simulink model "DV3A_String1_Diode"  (R2023b)
settings: Solver=VariableStepAuto  StartTime=0.0  StopTime=1  FixedStep=Ts_Power  MinStep=0.0025  RelTol=1e-4
PreLoadFcn:
  | Ts_Power=5e-4;
  | Slope_Vdc=1;
InitFcn:
  | Ts_Power=50e-6;
  | Tc=1e-5;%break algebraic loop time constant
StopFcn:
  | if exist('I','var') && exist('V','var')
  |    figure(1)
  |    clf
  |    n=find(I>=0);
  |    n=n(end);
  |    Vglobal=V(1:n);
  |    Iglobal=I(1:n);
  | 
  | 
  |    Pglobal=Vglobal.*Iglobal;
  |    n=find(Pglobal==max(Pglobal));
  |    Pmax=Pglobal(n);
  |    Vmp=Vglobal(n);
  |    Imp=Iglobal(n);
  | 
  | 
  |    subplot(211)
  |    plot(Vglobal, Iglobal,Vmp,Imp,'or')
  |    ylabel('Current (A)')
  |    title(sprintf('Global I-V & P-V characteristics\n %s' ,ModuleName))
  | 
  | 
  |    subplot(212)
  |    plot(Vglobal, Pglobal,Vmp,Pmax,'or')
  |    ylabel('Power (W)')
  |    xlabel('Voltage (V)')
  | end
model workspace (MAT data in the model file):
  slope_Vdc = 3.0848387096
values from neighbouring files (symbols this model uses):
  Slope_Vdc_string1 = Slope_Vdc_string(1)    [totPower.m]
libraries: spsPVArrayLib x121, spsVariableResistorLib x121, spsDiodeLib x24, spsCurrentMeasurementLib x1, spsVoltageMeasurementLib x1, spsControlledVoltageSourceLib x1, simulink x1, spspowerguiLib x1
(part 1 of 7)
settings Model: Creator=MathWorks  LastModifiedBy=IT
settings SolverCC: AlgebraicLoopSolver=LineSearch
settings DataIOCC: ExternalInput=[]  LimitDataPoints=on  LoadExternalInput=on  SaveFormat=Array  SaveOutput=off  SignalLogging=off  DSMLogging=off  SaveTime=off  ReturnWorkspaceOutputs=off
settings OptimizationCC: ExpressionDepthLimit=2147483647  LifeSpan=inf
settings DebuggingCC: UnderspecifiedInitializationDetection=Classic  MergeDetectMultiDrivingBlocksExec=none  SolverPrmCheckMsg=warning  FcnCallInpInsideContextMsg=warning  UnconnectedInputMsg=warning  UnconnectedOutputMsg=warning  UnconnectedLineMsg=warning  AllowSymbolicDim=off  StateNameClashWarn=warning  SFUnexpectedBacktrackingDiag=warning  SFNoUnconditionalDefaultTransitionDiag=warning  SFExecutionAtInitializationDiag=none  ArithmeticOperatorsInVariantConditions=warning
settings HardwareCC: ProdBitPerPointer=32  ProdBitPerSizeT=32  ProdBitPerPtrDiffT=32  ProdLargestAtomicFloat=None  ProdIntDivRoundTo=Undefined  ProdEndianess=Unspecified  ProdWordSize=32  ProdHWDeviceType=32-bit Generic
settings ModelReferenceCC: EnableRefExpFcnMdlSchedulingChecks=on  PropagateSignalLabelsOutOfModel=off
settings SFSimCC: SimUseLocalCustomCode=off  CustomCodeUndefinedFunction=UseInterfaceOnly
settings RTWCC: RTWUseLocalCustomCode=off  DLArmComputeVersion=19.05
settings CodeAppCC: StateflowObjectComments=on
settings GRTTargetCC: TargetLangStandard=C89/C90 (ANSI)  CombineOutputUpdateFcns=off  GRTInterface=on
settings ConfigComp: CovMetricSettings=dw  CovSaveCumulativeToWorkspaceVar=on  CovSaveSingleToWorkspaceVar=on  CovExternalEMLEnable=off  CovSFcnEnable=off
settings SimscapeCC: SimscapeNormalizeSystem=off

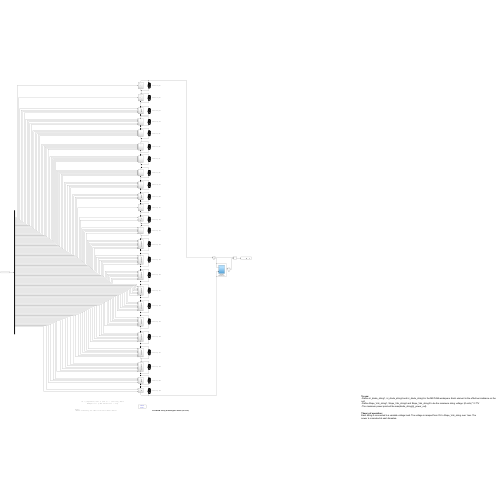
[thumbnail: Simulink's stored preview of the top-level diagram]
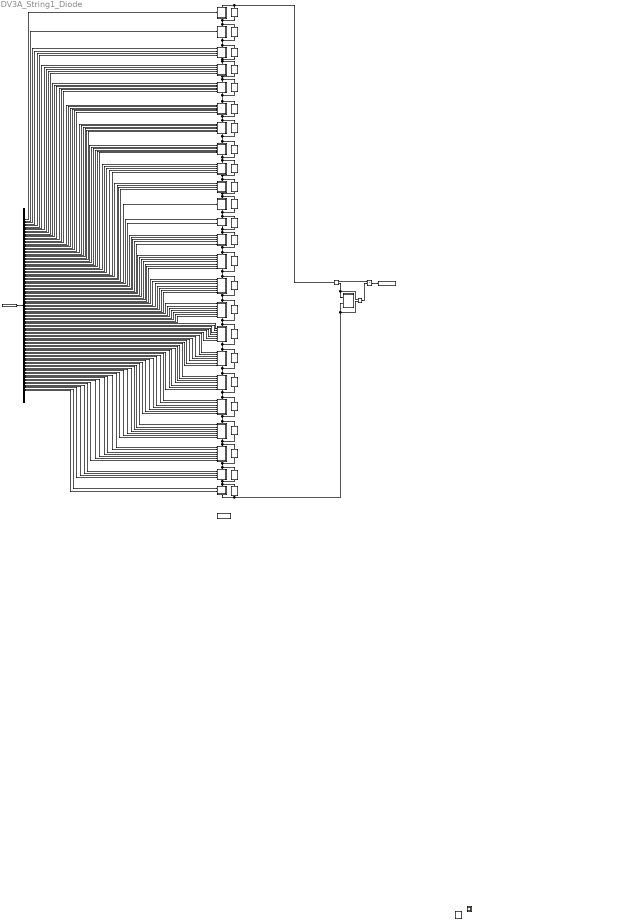
== system DV3A_String1_Diode ==
  note: irr = [(required 0) (cell 1) (cell 2) ... (cell 121)], W/m^2
  note: Notes:
      | -Within a substring, the order of the cells doesn't matter
  note: Final DV3B - String #1 with bypass diodes (121 cells)
  note: Example: irr = [0 800 700 242 573.3 ... 473]
  note: To use:
      | -Define irr_diode_string1, irr_diode_string2 and irr_diode_string3 in the MATLAB workspace. Each element is the effective irradiance on the cell
      | -Define Slope_Vdc_string1, Slope_Vdc_string2 and Slope_Vdc_string3 to be the maximum string voltage: (# cells) * 0.77V
      | -The maximum power point will be max(diode_string[n]_power_out )
  note: Theory of operation:
      | Each string is connected to a variable voltage load. The voltage is ramped from 0V to Slope_Vdc_string over 1sec. The power is computed at each timestep.
  note: Substring #1
  note: Substring #2
  note: Substring #3
  note: Substring #4
  note: Substring #5
  note: Substring #6
  note: Substring #8
  note: Substring #7
  note: Substring #9
  note: Substring #10
  note: Substring #11
  note: Substring #12
  note: Substring #13
  note: Substring #14
  note: Substring #15
  note: Substring #17
  note: Substring #16
  note: Substring #19
  note: Substring #18
  note: Substring #20
  note: Substring #21
  note: Substring #22
  note: Substring #23
  note: Substring #24
  Bypass Diode {1..11,21..33} (24 alike) : spsDiodeLib/Diode  Ron=0.00333333  Lon=0  Vf=0.01993333134  IC=0  UseSnubber=off  Rs=1000000000  Cs=250e-15  Measurements=off
  Demux2 : Demux  Outputs=121
  From Workspace2 : FromWorkspace  VariableName=irr_diode_string_String1
  I1 : spsCurrentMeasurementLib/Current Measurement  PhasorSimulation=off  OutputType=Complex  PSBequivalent=0
  Product2 : Product
  Subsystem1 : Subsystem
      settings: PortSchema="{\"entries\":[{\"content\":{\"sides\":[{\"content\":{\"connectorIds\":[\"In1\",\"In2\",\"In3\",\"In4\",\"In5\",\"In6\",\"In7\"]},\"type\":\"ConnectorPlacement.EquallySpacedRectSide\",\"uuid\":\"ec6071b1-e44d-45a4-9204-34cda7b2c9be\"},{\"content\":{\"connectorIds\":[],\"side\":\"RIGHT\"},\"type\":\"ConnectorPlacement.EquallySpacedRectSide\",\"uuid\":\"8ac2ba72-278d-4942-985d-63a53d830fa7\"},{\"content\":{\"connectorIds\":[\"LConn1\"],\"side\":\"TOP\"},\"type\":\"ConnectorPlacement.EquallySpacedRectSide\",\"uuid\":\"91abef48-6106-4bba-9094-b5b4c6d4927b\"},{\"content\":{\"connectorIds\":[\"RConn1\"],\"side\":\"BOTTOM\"},\"type\":\"ConnectorPlacement.EquallySpacedRectSide\",\"uuid\":\"2339e630-2664-445f-8cd2-24ead5b760e5\"}]},\"type\":\"ConnectorPlacement.EquallySpacedConnector\",\"uuid\":\"6b30c10d-3aac-43c1-96cb-d205f04f2f88\"}],\"packageUris\":[\"http://schema.mathworks.com/mf0/Connector/R2020b\"],\"version\":\"1.0\"}"
  Subsystem10 : Subsystem
      settings: PortSchema="{\"entries\":[{\"content\":{\"sides\":[{\"content\":{\"connectorIds\":[\"In1\",\"In2\",\"In3\",\"In4\"]},\"type\":\"ConnectorPlacement.EquallySpacedRectSide\",\"uuid\":\"ec6071b1-e44d-45a4-9204-34cda7b2c9be\"},{\"content\":{\"connectorIds\":[],\"side\":\"RIGHT\"},\"type\":\"ConnectorPlacement.EquallySpacedRectSide\",\"uuid\":\"8ac2ba72-278d-4942-985d-63a53d830fa7\"},{\"content\":{\"connectorIds\":[\"LConn1\"],\"side\":\"TOP\"},\"type\":\"ConnectorPlacement.EquallySpacedRectSide\",\"uuid\":\"91abef48-6106-4bba-9094-b5b4c6d4927b\"},{\"content\":{\"connectorIds\":[\"RConn1\"],\"side\":\"BOTTOM\"},\"type\":\"ConnectorPlacement.EquallySpacedRectSide\",\"uuid\":\"2339e630-2664-445f-8cd2-24ead5b760e5\"}]},\"type\":\"ConnectorPlacement.EquallySpacedConnector\",\"uuid\":\"6b30c10d-3aac-43c1-96cb-d205f04f2f88\"}],\"packageUris\":[\"http://schema.mathworks.com/mf0/Connector/R2020b\"],\"version\":\"1.0\"}"
  Subsystem11 : Subsystem
      settings: PortSchema="{\"entries\":[{\"content\":{\"sides\":[{\"content\":{\"connectorIds\":[\"In1\",\"In2\"]},\"type\":\"ConnectorPlacement.EquallySpacedRectSide\",\"uuid\":\"ec6071b1-e44d-45a4-9204-34cda7b2c9be\"},{\"content\":{\"connectorIds\":[],\"side\":\"RIGHT\"},\"type\":\"ConnectorPlacement.EquallySpacedRectSide\",\"uuid\":\"8ac2ba72-278d-4942-985d-63a53d830fa7\"},{\"content\":{\"connectorIds\":[\"LConn1\"],\"side\":\"TOP\"},\"type\":\"ConnectorPlacement.EquallySpacedRectSide\",\"uuid\":\"91abef48-6106-4bba-9094-b5b4c6d4927b\"},{\"content\":{\"connectorIds\":[\"RConn1\"],\"side\":\"BOTTOM\"},\"type\":\"ConnectorPlacement.EquallySpacedRectSide\",\"uuid\":\"2339e630-2664-445f-8cd2-24ead5b760e5\"}]},\"type\":\"ConnectorPlacement.EquallySpacedConnector\",\"uuid\":\"6b30c10d-3aac-43c1-96cb-d205f04f2f88\"}],\"packageUris\":[\"http://schema.mathworks.com/mf0/Connector/R2020b\"],\"version\":\"1.0\"}"
  Subsystem2 : Subsystem
      settings: PortSchema="{\"entries\":[{\"content\":{\"sides\":[{\"content\":{\"connectorIds\":[\"In1\",\"In2\",\"In3\",\"In4\",\"In5\",\"In6\",\"In7\"]},\"type\":\"ConnectorPlacement.EquallySpacedRectSide\",\"uuid\":\"ec6071b1-e44d-45a4-9204-34cda7b2c9be\"},{\"content\":{\"connectorIds\":[],\"side\":\"RIGHT\"},\"type\":\"ConnectorPlacement.EquallySpacedRectSide\",\"uuid\":\"8ac2ba72-278d-4942-985d-63a53d830fa7\"},{\"content\":{\"connectorIds\":[\"LConn1\"],\"side\":\"TOP\"},\"type\":\"ConnectorPlacement.EquallySpacedRectSide\",\"uuid\":\"91abef48-6106-4bba-9094-b5b4c6d4927b\"},{\"content\":{\"connectorIds\":[\"RConn1\"],\"side\":\"BOTTOM\"},\"type\":\"ConnectorPlacement.EquallySpacedRectSide\",\"uuid\":\"2339e630-2664-445f-8cd2-24ead5b760e5\"}]},\"type\":\"ConnectorPlacement.EquallySpacedConnector\",\"uuid\":\"6b30c10d-3aac-43c1-96cb-d205f04f2f88\"}],\"packageUris\":[\"http://schema.mathworks.com/mf0/Connector/R2020b\"],\"version\":\"1.0\"}"
  Subsystem21 : Subsystem
      settings: PortSchema="{\"entries\":[{\"content\":{\"sides\":[{\"content\":{\"connectorIds\":[\"In1\"]},\"type\":\"ConnectorPlacement.EquallySpacedRectSide\",\"uuid\":\"ec6071b1-e44d-45a4-9204-34cda7b2c9be\"},{\"content\":{\"side\":\"RIGHT\"},\"type\":\"ConnectorPlacement.EquallySpacedRectSide\",\"uuid\":\"8ac2ba72-278d-4942-985d-63a53d830fa7\"},{\"content\":{\"connectorIds\":[\"LConn1\"],\"side\":\"TOP\"},\"type\":\"ConnectorPlacement.EquallySpacedRectSide\",\"uuid\":\"91abef48-6106-4bba-9094-b5b4c6d4927b\"},{\"content\":{\"connectorIds\":[\"RConn1\"],\"side\":\"BOTTOM\"},\"type\":\"ConnectorPlacement.EquallySpacedRectSide\",\"uuid\":\"2339e630-2664-445f-8cd2-24ead5b760e5\"}]},\"type\":\"ConnectorPlacement.EquallySpacedConnector\",\"uuid\":\"6b30c10d-3aac-43c1-96cb-d205f04f2f88\"}],\"packageUris\":[\"http://schema.mathworks.com/mf0/Connector/R2020b\"],\"version\":\"1.0\"}"
  Subsystem22 : Subsystem
      settings: PortSchema="{\"entries\":[{\"content\":{\"sides\":[{\"content\":{\"connectorIds\":[\"In1\"]},\"type\":\"ConnectorPlacement.EquallySpacedRectSide\",\"uuid\":\"ec6071b1-e44d-45a4-9204-34cda7b2c9be\"},{\"content\":{\"side\":\"RIGHT\"},\"type\":\"ConnectorPlacement.EquallySpacedRectSide\",\"uuid\":\"8ac2ba72-278d-4942-985d-63a53d830fa7\"},{\"content\":{\"connectorIds\":[\"LConn1\"],\"side\":\"TOP\"},\"type\":\"ConnectorPlacement.EquallySpacedRectSide\",\"uuid\":\"91abef48-6106-4bba-9094-b5b4c6d4927b\"},{\"content\":{\"connectorIds\":[\"RConn1\"],\"side\":\"BOTTOM\"},\"type\":\"ConnectorPlacement.EquallySpacedRectSide\",\"uuid\":\"2339e630-2664-445f-8cd2-24ead5b760e5\"}]},\"type\":\"ConnectorPlacement.EquallySpacedConnector\",\"uuid\":\"6b30c10d-3aac-43c1-96cb-d205f04f2f88\"}],\"packageUris\":[\"http://schema.mathworks.com/mf0/Connector/R2020b\"],\"version\":\"1.0\"}"
  Subsystem23 : Subsystem
      settings: PortSchema="{\"entries\":[{\"content\":{\"sides\":[{\"content\":{\"connectorIds\":[\"In1\",\"In2\",\"In3\",\"In4\"]},\"type\":\"ConnectorPlacement.EquallySpacedRectSide\",\"uuid\":\"ec6071b1-e44d-45a4-9204-34cda7b2c9be\"},{\"content\":{\"connectorIds\":[],\"side\":\"RIGHT\"},\"type\":\"ConnectorPlacement.EquallySpacedRectSide\",\"uuid\":\"8ac2ba72-278d-4942-985d-63a53d830fa7\"},{\"content\":{\"connectorIds\":[\"LConn1\"],\"side\":\"TOP\"},\"type\":\"ConnectorPlacement.EquallySpacedRectSide\",\"uuid\":\"91abef48-6106-4bba-9094-b5b4c6d4927b\"},{\"content\":{\"connectorIds\":[\"RConn1\"],\"side\":\"BOTTOM\"},\"type\":\"ConnectorPlacement.EquallySpacedRectSide\",\"uuid\":\"2339e630-2664-445f-8cd2-24ead5b760e5\"}]},\"type\":\"ConnectorPlacement.EquallySpacedConnector\",\"uuid\":\"6b30c10d-3aac-43c1-96cb-d205f04f2f88\"}],\"packageUris\":[\"http://schema.mathworks.com/mf0/Connector/R2020b\"],\"version\":\"1.0\"}"
  Subsystem24 : Subsystem
      settings: PortSchema="{\"entries\":[{\"content\":{\"sides\":[{\"content\":{\"connectorIds\":[\"In1\",\"In2\",\"In3\",\"In4\",\"In5\"]},\"type\":\"ConnectorPlacement.EquallySpacedRectSide\",\"uuid\":\"ec6071b1-e44d-45a4-9204-34cda7b2c9be\"},{\"content\":{\"side\":\"RIGHT\"},\"type\":\"ConnectorPlacement.EquallySpacedRectSide\",\"uuid\":\"8ac2ba72-278d-4942-985d-63a53d830fa7\"},{\"content\":{\"connectorIds\":[\"LConn1\"],\"side\":\"TOP\"},\"type\":\"ConnectorPlacement.EquallySpacedRectSide\",\"uuid\":\"91abef48-6106-4bba-9094-b5b4c6d4927b\"},{\"content\":{\"connectorIds\":[\"RConn1\"],\"side\":\"BOTTOM\"},\"type\":\"ConnectorPlacement.EquallySpacedRectSide\",\"uuid\":\"2339e630-2664-445f-8cd2-24ead5b760e5\"}]},\"type\":\"ConnectorPlacement.EquallySpacedConnector\",\"uuid\":\"6b30c10d-3aac-43c1-96cb-d205f04f2f88\"}],\"packageUris\":[\"http://schema.mathworks.com/mf0/Connector/R2020b\"],\"version\":\"1.0\"}"
  Subsystem25 : Subsystem
      settings: PortSchema="{\"entries\":[{\"content\":{\"sides\":[{\"content\":{\"connectorIds\":[\"In1\",\"In2\",\"In3\",\"In4\",\"In5\",\"In6\"]},\"type\":\"ConnectorPlacement.EquallySpacedRectSide\",\"uuid\":\"ec6071b1-e44d-45a4-9204-34cda7b2c9be\"},{\"content\":{\"side\":\"RIGHT\"},\"type\":\"ConnectorPlacement.EquallySpacedRectSide\",\"uuid\":\"8ac2ba72-278d-4942-985d-63a53d830fa7\"},{\"content\":{\"connectorIds\":[\"LConn1\"],\"side\":\"TOP\"},\"type\":\"ConnectorPlacement.EquallySpacedRectSide\",\"uuid\":\"91abef48-6106-4bba-9094-b5b4c6d4927b\"},{\"content\":{\"connectorIds\":[\"RConn1\"],\"side\":\"BOTTOM\"},\"type\":\"ConnectorPlacement.EquallySpacedRectSide\",\"uuid\":\"2339e630-2664-445f-8cd2-24ead5b760e5\"}]},\"type\":\"ConnectorPlacement.EquallySpacedConnector\",\"uuid\":\"6b30c10d-3aac-43c1-96cb-d205f04f2f88\"}],\"packageUris\":[\"http://schema.mathworks.com/mf0/Connector/R2020b\"],\"version\":\"1.0\"}"
  Subsystem26 : Subsystem
      settings: PortSchema="{\"entries\":[{\"content\":{\"sides\":[{\"content\":{\"connectorIds\":[\"In1\",\"In2\",\"In3\",\"In4\",\"In5\",\"In6\"]},\"type\":\"ConnectorPlacement.EquallySpacedRectSide\",\"uuid\":\"ec6071b1-e44d-45a4-9204-34cda7b2c9be\"},{\"content\":{\"side\":\"RIGHT\"},\"type\":\"ConnectorPlacement.EquallySpacedRectSide\",\"uuid\":\"8ac2ba72-278d-4942-985d-63a53d830fa7\"},{\"content\":{\"connectorIds\":[\"LConn1\"],\"side\":\"TOP\"},\"type\":\"ConnectorPlacement.EquallySpacedRectSide\",\"uuid\":\"91abef48-6106-4bba-9094-b5b4c6d4927b\"},{\"content\":{\"connectorIds\":[\"RConn1\"],\"side\":\"BOTTOM\"},\"type\":\"ConnectorPlacement.EquallySpacedRectSide\",\"uuid\":\"2339e630-2664-445f-8cd2-24ead5b760e5\"}]},\"type\":\"ConnectorPlacement.EquallySpacedConnector\",\"uuid\":\"6b30c10d-3aac-43c1-96cb-d205f04f2f88\"}],\"packageUris\":[\"http://schema.mathworks.com/mf0/Connector/R2020b\"],\"version\":\"1.0\"}"
  Subsystem27 : Subsystem
      settings: PortSchema="{\"entries\":[{\"content\":{\"sides\":[{\"content\":{\"connectorIds\":[\"In1\",\"In2\",\"In3\",\"In4\",\"In5\",\"In6\"]},\"type\":\"ConnectorPlacement.EquallySpacedRectSide\",\"uuid\":\"ec6071b1-e44d-45a4-9204-34cda7b2c9be\"},{\"content\":{\"side\":\"RIGHT\"},\"type\":\"ConnectorPlacement.EquallySpacedRectSide\",\"uuid\":\"8ac2ba72-278d-4942-985d-63a53d830fa7\"},{\"content\":{\"connectorIds\":[\"LConn1\"],\"side\":\"TOP\"},\"type\":\"ConnectorPlacement.EquallySpacedRectSide\",\"uuid\":\"91abef48-6106-4bba-9094-b5b4c6d4927b\"},{\"content\":{\"connectorIds\":[\"RConn1\"],\"side\":\"BOTTOM\"},\"type\":\"ConnectorPlacement.EquallySpacedRectSide\",\"uuid\":\"2339e630-2664-445f-8cd2-24ead5b760e5\"}]},\"type\":\"ConnectorPlacement.EquallySpacedConnector\",\"uuid\":\"6b30c10d-3aac-43c1-96cb-d205f04f2f88\"}],\"packageUris\":[\"http://schema.mathworks.com/mf0/Connector/R2020b\"],\"version\":\"1.0\"}"
  Subsystem28 : Subsystem
      settings: PortSchema="{\"entries\":[{\"content\":{\"sides\":[{\"content\":{\"connectorIds\":[\"In1\",\"In2\",\"In3\",\"In4\",\"In5\"]},\"type\":\"ConnectorPlacement.EquallySpacedRectSide\",\"uuid\":\"ec6071b1-e44d-45a4-9204-34cda7b2c9be\"},{\"content\":{\"side\":\"RIGHT\"},\"type\":\"ConnectorPlacement.EquallySpacedRectSide\",\"uuid\":\"8ac2ba72-278d-4942-985d-63a53d830fa7\"},{\"content\":{\"connectorIds\":[\"LConn1\"],\"side\":\"TOP\"},\"type\":\"ConnectorPlacement.EquallySpacedRectSide\",\"uuid\":\"91abef48-6106-4bba-9094-b5b4c6d4927b\"},{\"content\":{\"connectorIds\":[\"RConn1\"],\"side\":\"BOTTOM\"},\"type\":\"ConnectorPlacement.EquallySpacedRectSide\",\"uuid\":\"2339e630-2664-445f-8cd2-24ead5b760e5\"}]},\"type\":\"ConnectorPlacement.EquallySpacedConnector\",\"uuid\":\"6b30c10d-3aac-43c1-96cb-d205f04f2f88\"}],\"packageUris\":[\"http://schema.mathworks.com/mf0/Connector/R2020b\"],\"version\":\"1.0\"}"
  Subsystem29 : Subsystem
      settings: PortSchema="{\"entries\":[{\"content\":{\"sides\":[{\"content\":{\"connectorIds\":[\"In1\",\"In2\",\"In3\",\"In4\",\"In5\",\"In6\"]},\"type\":\"ConnectorPlacement.EquallySpacedRectSide\",\"uuid\":\"ec6071b1-e44d-45a4-9204-34cda7b2c9be\"},{\"content\":{\"side\":\"RIGHT\"},\"type\":\"ConnectorPlacement.EquallySpacedRectSide\",\"uuid\":\"8ac2ba72-278d-4942-985d-63a53d830fa7\"},{\"content\":{\"connectorIds\":[\"LConn1\"],\"side\":\"TOP\"},\"type\":\"ConnectorPlacement.EquallySpacedRectSide\",\"uuid\":\"91abef48-6106-4bba-9094-b5b4c6d4927b\"},{\"content\":{\"connectorIds\":[\"RConn1\"],\"side\":\"BOTTOM\"},\"type\":\"ConnectorPlacement.EquallySpacedRectSide\",\"uuid\":\"2339e630-2664-445f-8cd2-24ead5b760e5\"}]},\"type\":\"ConnectorPlacement.EquallySpacedConnector\",\"uuid\":\"6b30c10d-3aac-43c1-96cb-d205f04f2f88\"}],\"packageUris\":[\"http://schema.mathworks.com/mf0/Connector/R2020b\"],\"version\":\"1.0\"}"
  Subsystem3 : Subsystem
      settings: PortSchema="{\"entries\":[{\"content\":{\"sides\":[{\"content\":{\"connectorIds\":[\"In1\",\"In2\",\"In3\",\"In4\",\"In5\",\"In6\",\"In7\"]},\"type\":\"ConnectorPlacement.EquallySpacedRectSide\",\"uuid\":\"ec6071b1-e44d-45a4-9204-34cda7b2c9be\"},{\"content\":{\"connectorIds\":[],\"side\":\"RIGHT\"},\"type\":\"ConnectorPlacement.EquallySpacedRectSide\",\"uuid\":\"8ac2ba72-278d-4942-985d-63a53d830fa7\"},{\"content\":{\"connectorIds\":[\"LConn1\"],\"side\":\"TOP\"},\"type\":\"ConnectorPlacement.EquallySpacedRectSide\",\"uuid\":\"91abef48-6106-4bba-9094-b5b4c6d4927b\"},{\"content\":{\"connectorIds\":[\"RConn1\"],\"side\":\"BOTTOM\"},\"type\":\"ConnectorPlacement.EquallySpacedRectSide\",\"uuid\":\"2339e630-2664-445f-8cd2-24ead5b760e5\"}]},\"type\":\"ConnectorPlacement.EquallySpacedConnector\",\"uuid\":\"6b30c10d-3aac-43c1-96cb-d205f04f2f88\"}],\"packageUris\":[\"http://schema.mathworks.com/mf0/Connector/R2020b\"],\"version\":\"1.0\"}"
  Subsystem30 : Subsystem
      settings: PortSchema="{\"entries\":[{\"content\":{\"sides\":[{\"content\":{\"connectorIds\":[\"In1\",\"In2\",\"In3\",\"In4\"]},\"type\":\"ConnectorPlacement.EquallySpacedRectSide\",\"uuid\":\"ec6071b1-e44d-45a4-9204-34cda7b2c9be\"},{\"content\":{\"connectorIds\":[],\"side\":\"RIGHT\"},\"type\":\"ConnectorPlacement.EquallySpacedRectSide\",\"uuid\":\"8ac2ba72-278d-4942-985d-63a53d830fa7\"},{\"content\":{\"connectorIds\":[\"LConn1\"],\"side\":\"TOP\"},\"type\":\"ConnectorPlacement.EquallySpacedRectSide\",\"uuid\":\"91abef48-6106-4bba-9094-b5b4c6d4927b\"},{\"content\":{\"connectorIds\":[\"RConn1\"],\"side\":\"BOTTOM\"},\"type\":\"ConnectorPlacement.EquallySpacedRectSide\",\"uuid\":\"2339e630-2664-445f-8cd2-24ead5b760e5\"}]},\"type\":\"ConnectorPlacement.EquallySpacedConnector\",\"uuid\":\"6b30c10d-3aac-43c1-96cb-d205f04f2f88\"}],\"packageUris\":[\"http://schema.mathworks.com/mf0/Connector/R2020b\"],\"version\":\"1.0\"}"
  Subsystem31 : Subsystem
      settings: PortSchema="{\"entries\":[{\"content\":{\"sides\":[{\"content\":{\"connectorIds\":[\"In1\"]},\"type\":\"ConnectorPlacement.EquallySpacedRectSide\",\"uuid\":\"ec6071b1-e44d-45a4-9204-34cda7b2c9be\"},{\"content\":{\"side\":\"RIGHT\"},\"type\":\"ConnectorPlacement.EquallySpacedRectSide\",\"uuid\":\"8ac2ba72-278d-4942-985d-63a53d830fa7\"},{\"content\":{\"connectorIds\":[\"LConn1\"],\"side\":\"TOP\"},\"type\":\"ConnectorPlacement.EquallySpacedRectSide\",\"uuid\":\"91abef48-6106-4bba-9094-b5b4c6d4927b\"},{\"content\":{\"connectorIds\":[\"RConn1\"],\"side\":\"BOTTOM\"},\"type\":\"ConnectorPlacement.EquallySpacedRectSide\",\"uuid\":\"2339e630-2664-445f-8cd2-24ead5b760e5\"}]},\"type\":\"ConnectorPlacement.EquallySpacedConnector\",\"uuid\":\"6b30c10d-3aac-43c1-96cb-d205f04f2f88\"}],\"packageUris\":[\"http://schema.mathworks.com/mf0/Connector/R2020b\"],\"version\":\"1.0\"}"
  Subsystem32 : Subsystem
      settings: PortSchema="{\"entries\":[{\"content\":{\"sides\":[{\"content\":{\"connectorIds\":[\"In1\",\"In2\"]},\"type\":\"ConnectorPlacement.EquallySpacedRectSide\",\"uuid\":\"ec6071b1-e44d-45a4-9204-34cda7b2c9be\"},{\"content\":{\"connectorIds\":[],\"side\":\"RIGHT\"},\"type\":\"ConnectorPlacement.EquallySpacedRectSide\",\"uuid\":\"8ac2ba72-278d-4942-985d-63a53d830fa7\"},{\"content\":{\"connectorIds\":[\"LConn1\"],\"side\":\"TOP\"},\"type\":\"ConnectorPlacement.EquallySpacedRectSide\",\"uuid\":\"91abef48-6106-4bba-9094-b5b4c6d4927b\"},{\"content\":{\"connectorIds\":[\"RConn1\"],\"side\":\"BOTTOM\"},\"type\":\"ConnectorPlacement.EquallySpacedRectSide\",\"uuid\":\"2339e630-2664-445f-8cd2-24ead5b760e5\"}]},\"type\":\"ConnectorPlacement.EquallySpacedConnector\",\"uuid\":\"6b30c10d-3aac-43c1-96cb-d205f04f2f88\"}],\"packageUris\":[\"http://schema.mathworks.com/mf0/Connector/R2020b\"],\"version\":\"1.0\"}"
  Subsystem33 : Subsystem
      settings: PortSchema="{\"entries\":[{\"content\":{\"sides\":[{\"content\":{\"connectorIds\":[\"In1\",\"In2\",\"In3\",\"In4\",\"In5\"]},\"type\":\"ConnectorPlacement.EquallySpacedRectSide\",\"uuid\":\"ec6071b1-e44d-45a4-9204-34cda7b2c9be\"},{\"content\":{\"side\":\"RIGHT\"},\"type\":\"ConnectorPlacement.EquallySpacedRectSide\",\"uuid\":\"8ac2ba72-278d-4942-985d-63a53d830fa7\"},{\"content\":{\"connectorIds\":[\"LConn1\"],\"side\":\"TOP\"},\"type\":\"ConnectorPlacement.EquallySpacedRectSide\",\"uuid\":\"91abef48-6106-4bba-9094-b5b4c6d4927b\"},{\"content\":{\"connectorIds\":[\"RConn1\"],\"side\":\"BOTTOM\"},\"type\":\"ConnectorPlacement.EquallySpacedRectSide\",\"uuid\":\"2339e630-2664-445f-8cd2-24ead5b760e5\"}]},\"type\":\"ConnectorPlacement.EquallySpacedConnector\",\"uuid\":\"6b30c10d-3aac-43c1-96cb-d205f04f2f88\"}],\"packageUris\":[\"http://schema.mathworks.com/mf0/Connector/R2020b\"],\"version\":\"1.0\"}"
  Subsystem4 : Subsystem
      settings: PortSchema="{\"entries\":[{\"content\":{\"sides\":[{\"content\":{\"connectorIds\":[\"In1\",\"In2\",\"In3\",\"In4\",\"In5\",\"In6\",\"In7\"]},\"type\":\"ConnectorPlacement.EquallySpacedRectSide\",\"uuid\":\"ec6071b1-e44d-45a4-9204-34cda7b2c9be\"},{\"content\":{\"connectorIds\":[],\"side\":\"RIGHT\"},\"type\":\"ConnectorPlacement.EquallySpacedRectSide\",\"uuid\":\"8ac2ba72-278d-4942-985d-63a53d830fa7\"},{\"content\":{\"connectorIds\":[\"LConn1\"],\"side\":\"TOP\"},\"type\":\"ConnectorPlacement.EquallySpacedRectSide\",\"uuid\":\"91abef48-6106-4bba-9094-b5b4c6d4927b\"},{\"content\":{\"connectorIds\":[\"RConn1\"],\"side\":\"BOTTOM\"},\"type\":\"ConnectorPlacement.EquallySpacedRectSide\",\"uuid\":\"2339e630-2664-445f-8cd2-24ead5b760e5\"}]},\"type\":\"ConnectorPlacement.EquallySpacedConnector\",\"uuid\":\"6b30c10d-3aac-43c1-96cb-d205f04f2f88\"}],\"packageUris\":[\"http://schema.mathworks.com/mf0/Connector/R2020b\"],\"version\":\"1.0\"}"
  Subsystem5 : Subsystem
      settings: PortSchema="{\"entries\":[{\"content\":{\"sides\":[{\"content\":{\"connectorIds\":[\"In1\",\"In2\",\"In3\",\"In4\",\"In5\",\"In6\",\"In7\"]},\"type\":\"ConnectorPlacement.EquallySpacedRectSide\",\"uuid\":\"ec6071b1-e44d-45a4-9204-34cda7b2c9be\"},{\"content\":{\"connectorIds\":[],\"side\":\"RIGHT\"},\"type\":\"ConnectorPlacement.EquallySpacedRectSide\",\"uuid\":\"8ac2ba72-278d-4942-985d-63a53d830fa7\"},{\"content\":{\"connectorIds\":[\"LConn1\"],\"side\":\"TOP\"},\"type\":\"ConnectorPlacement.EquallySpacedRectSide\",\"uuid\":\"91abef48-6106-4bba-9094-b5b4c6d4927b\"},{\"content\":{\"connectorIds\":[\"RConn1\"],\"side\":\"BOTTOM\"},\"type\":\"ConnectorPlacement.EquallySpacedRectSide\",\"uuid\":\"2339e630-2664-445f-8cd2-24ead5b760e5\"}]},\"type\":\"ConnectorPlacement.EquallySpacedConnector\",\"uuid\":\"6b30c10d-3aac-43c1-96cb-d205f04f2f88\"}],\"packageUris\":[\"http://schema.mathworks.com/mf0/Connector/R2020b\"],\"version\":\"1.0\"}"
  Subsystem6 : Subsystem
      settings: PortSchema="{\"entries\":[{\"content\":{\"sides\":[{\"content\":{\"connectorIds\":[\"In1\",\"In2\",\"In3\",\"In4\",\"In5\",\"In6\",\"In7\"]},\"type\":\"ConnectorPlacement.EquallySpacedRectSide\",\"uuid\":\"ec6071b1-e44d-45a4-9204-34cda7b2c9be\"},{\"content\":{\"connectorIds\":[],\"side\":\"RIGHT\"},\"type\":\"ConnectorPlacement.EquallySpacedRectSide\",\"uuid\":\"8ac2ba72-278d-4942-985d-63a53d830fa7\"},{\"content\":{\"connectorIds\":[\"LConn1\"],\"side\":\"TOP\"},\"type\":\"ConnectorPlacement.EquallySpacedRectSide\",\"uuid\":\"91abef48-6106-4bba-9094-b5b4c6d4927b\"},{\"content\":{\"connectorIds\":[\"RConn1\"],\"side\":\"BOTTOM\"},\"type\":\"ConnectorPlacement.EquallySpacedRectSide\",\"uuid\":\"2339e630-2664-445f-8cd2-24ead5b760e5\"}]},\"type\":\"ConnectorPlacement.EquallySpacedConnector\",\"uuid\":\"6b30c10d-3aac-43c1-96cb-d205f04f2f88\"}],\"packageUris\":[\"http://schema.mathworks.com/mf0/Connector/R2020b\"],\"version\":\"1.0\"}"
  Subsystem7 : Subsystem
      settings: PortSchema="{\"entries\":[{\"content\":{\"sides\":[{\"content\":{\"connectorIds\":[\"In1\",\"In2\",\"In3\",\"In4\",\"In5\",\"In6\",\"In7\"]},\"type\":\"ConnectorPlacement.EquallySpacedRectSide\",\"uuid\":\"ec6071b1-e44d-45a4-9204-34cda7b2c9be\"},{\"content\":{\"connectorIds\":[],\"side\":\"RIGHT\"},\"type\":\"ConnectorPlacement.EquallySpacedRectSide\",\"uuid\":\"8ac2ba72-278d-4942-985d-63a53d830fa7\"},{\"content\":{\"connectorIds\":[\"LConn1\"],\"side\":\"TOP\"},\"type\":\"ConnectorPlacement.EquallySpacedRectSide\",\"uuid\":\"91abef48-6106-4bba-9094-b5b4c6d4927b\"},{\"content\":{\"connectorIds\":[\"RConn1\"],\"side\":\"BOTTOM\"},\"type\":\"ConnectorPlacement.EquallySpacedRectSide\",\"uuid\":\"2339e630-2664-445f-8cd2-24ead5b760e5\"}]},\"type\":\"ConnectorPlacement.EquallySpacedConnector\",\"uuid\":\"6b30c10d-3aac-43c1-96cb-d205f04f2f88\"}],\"packageUris\":[\"http://schema.mathworks.com/mf0/Connector/R2020b\"],\"version\":\"1.0\"}"
  Subsystem8 : Subsystem
      settings: PortSchema="{\"entries\":[{\"content\":{\"sides\":[{\"content\":{\"connectorIds\":[\"In1\",\"In2\",\"In3\",\"In4\",\"In5\",\"In6\",\"In7\"]},\"type\":\"ConnectorPlacement.EquallySpacedRectSide\",\"uuid\":\"ec6071b1-e44d-45a4-9204-34cda7b2c9be\"},{\"content\":{\"connectorIds\":[],\"side\":\"RIGHT\"},\"type\":\"ConnectorPlacement.EquallySpacedRectSide\",\"uuid\":\"8ac2ba72-278d-4942-985d-63a53d830fa7\"},{\"content\":{\"connectorIds\":[\"LConn1\"],\"side\":\"TOP\"},\"type\":\"ConnectorPlacement.EquallySpacedRectSide\",\"uuid\":\"91abef48-6106-4bba-9094-b5b4c6d4927b\"},{\"content\":{\"connectorIds\":[\"RConn1\"],\"side\":\"BOTTOM\"},\"type\":\"ConnectorPlacement.EquallySpacedRectSide\",\"uuid\":\"2339e630-2664-445f-8cd2-24ead5b760e5\"}]},\"type\":\"ConnectorPlacement.EquallySpacedConnector\",\"uuid\":\"6b30c10d-3aac-43c1-96cb-d205f04f2f88\"}],\"packageUris\":[\"http://schema.mathworks.com/mf0/Connector/R2020b\"],\"version\":\"1.0\"}"
  Subsystem9 : Subsystem
      settings: PortSchema="{\"entries\":[{\"content\":{\"sides\":[{\"content\":{\"connectorIds\":[\"In1\",\"In2\",\"In3\",\"In4\",\"In5\",\"In6\",\"In7\"]},\"type\":\"ConnectorPlacement.EquallySpacedRectSide\",\"uuid\":\"ec6071b1-e44d-45a4-9204-34cda7b2c9be\"},{\"content\":{\"connectorIds\":[],\"side\":\"RIGHT\"},\"type\":\"ConnectorPlacement.EquallySpacedRectSide\",\"uuid\":\"8ac2ba72-278d-4942-985d-63a53d830fa7\"},{\"content\":{\"connectorIds\":[\"LConn1\"],\"side\":\"TOP\"},\"type\":\"ConnectorPlacement.EquallySpacedRectSide\",\"uuid\":\"91abef48-6106-4bba-9094-b5b4c6d4927b\"},{\"content\":{\"connectorIds\":[\"RConn1\"],\"side\":\"BOTTOM\"},\"type\":\"ConnectorPlacement.EquallySpacedRectSide\",\"uuid\":\"2339e630-2664-445f-8cd2-24ead5b760e5\"}]},\"type\":\"ConnectorPlacement.EquallySpacedConnector\",\"uuid\":\"6b30c10d-3aac-43c1-96cb-d205f04f2f88\"}],\"packageUris\":[\"http://schema.mathworks.com/mf0/Connector/R2020b\"],\"version\":\"1.0\"}"
  To Workspace2 : ToWorkspace  VariableName=diode_string1_power_out  SampleTime=-1
      settings: Save2DSignal=2-D array (concatenate along first dimension)
  V1 : spsVoltageMeasurementLib/Voltage Measurement  PhasorSimulation=off  OutputType=Complex  PSBequivalent=0
  Variable DC Source1 : Subsystem
  powergui2 : spspowerguiLib/powergui  Priority=1  SimulationMode=Discrete  SampleTime=2.5e-3  frequency=60  Iterations=500  frequencyindice=0  Pbase=100e6  ErrMax=1e-4  UnitsV=kV  UnitsW=MW  buscounter=0  FunctionMessages=off  echomessages=off  EnableUseOfTLC=off  CurrentSourceSwitches=on  DisableSnubberDevices=on  DisableRonSwitches=off  DisableVfSwitches=off  DisplayEquations=off  AutomaticDiscreteSolvers=off  SolverType=Tustin/Backward Euler (TBE)  Interpol=off  ExternalGateDelay=off  methode=off  Ts=0  x0status=blocks  SPID=off  SwTol=0  HookPort=off  NonlinearTolerance=1e-4  nMaxIteration=1000  ContinueOnMaxIteration=off  RestoreLinks=warning  ResistiveCurrentMeasurement=off  Frange=[0:2:500]  Ylog=off  Xlog=on  ShowGrid=off  save=off  variable=ZData  structure=0  ZoomFFT=on  StartTime=0.0  cycles=1  DisplayStyle=1  fundamental=60  FreqAxis=off  MaxFrequency=1000  frequencyindicesteady=1  RmsSteady=1  display=off
  Array Plot : ArrayPlot  IOType=viewer  WindowPosition=[117.000000,351.000000,800.000000,450.000000,]  ScopeFrameLocation=window  AxesScaling=Manual  YLimits=[-1,1]
  Scope{,1..3} (4 alike) : Scope
  wires:
  V1/1 -> Product2/2
  Product2/1 -> To Workspace2/1
  I1/1 -> Product2/1
  From Workspace2/1 -> Demux2/1
  Demux2/1 -> Subsystem21/1(Irr)
  Demux2/2 -> Subsystem22/1(Irr)
  Demux2/3 -> Subsystem23/1(Irr)
  Demux2/4 -> Subsystem23/2(Irr1)
  Demux2/5 -> Subsystem23/3(Irr2)
  Demux2/6 -> Subsystem23/4(Irr3)
  Demux2/7 -> Subsystem24/1(Irr)
  Demux2/8 -> Subsystem24/2(Irr1)
  Demux2/9 -> Subsystem24/3(Irr2)
  Demux2/10 -> Subsystem24/4(Irr3)
  Demux2/11 -> Subsystem24/5(Irr4)
  Demux2/12 -> Subsystem29/1(Irr)
  Demux2/13 -> Subsystem29/2(Irr1)
  Demux2/14 -> Subsystem29/3(Irr3)
  Demux2/15 -> Subsystem29/4(Irr4)
  Demux2/16 -> Subsystem29/5(Irr2)
  Demux2/17 -> Subsystem29/6(Irr5)
  Demux2/18 -> Subsystem25/1(Irr)
  Demux2/19 -> Subsystem25/2(Irr1)
  Demux2/20 -> Subsystem25/3(Irr3)
  Demux2/21 -> Subsystem25/4(Irr4)
  Demux2/22 -> Subsystem25/5(Irr2)
  Demux2/23 -> Subsystem25/6(Irr5)
  Demux2/24 -> Subsystem27/1(Irr)
  Demux2/25 -> Subsystem27/2(Irr1)
  Demux2/26 -> Subsystem27/3(Irr3)
  Demux2/28 -> Subsystem27/5(Irr2)
  Demux2/27 -> Subsystem27/4(Irr4)
  Demux2/29 -> Subsystem27/6(Irr5)
  Demux2/30 -> Subsystem26/1(Irr)
  Demux2/31 -> Subsystem26/2(Irr1)
  Demux2/32 -> Subsystem26/3(Irr3)
  Demux2/33 -> Subsystem26/4(Irr4)
  Demux2/34 -> Subsystem26/5(Irr2)
  Demux2/35 -> Subsystem26/6(Irr5)
  Demux2/36 -> Subsystem28/1(Irr)
  Demux2/37 -> Subsystem28/2(Irr1)
  Demux2/38 -> Subsystem28/3(Irr2)
  Demux2/39 -> Subsystem28/4(Irr3)
  Demux2/40 -> Subsystem28/5(Irr4)
  Demux2/41 -> Subsystem30/1(Irr)
  Demux2/42 -> Subsystem30/2(Irr1)
  Demux2/43 -> Subsystem30/3(Irr2)
  Demux2/44 -> Subsystem30/4(Irr3)
  Demux2/45 -> Subsystem31/1(Irr)
  Demux2/46 -> Subsystem32/1(Irr)
  Demux2/47 -> Subsystem32/2(Irr1)
  Demux2/48 -> Subsystem33/1(Irr)
  Demux2/49 -> Subsystem33/2(Irr1)
  Demux2/50 -> Subsystem33/3(Irr2)
  Demux2/51 -> Subsystem33/4(Irr3)
  Demux2/52 -> Subsystem33/5(Irr4)
  Demux2/53 -> Subsystem1/1(Irr)
  Demux2/54 -> Subsystem1/2(Irr1)
  Demux2/55 -> Subsystem1/3(Irr2)
  Demux2/56 -> Subsystem1/4(Irr3)
  Demux2/57 -> Subsystem1/5(Irr4)
  Demux2/58 -> Subsystem1/6(Irr5)
  Demux2/59 -> Subsystem1/7(Irr6)
  Demux2/60 -> Subsystem2/1(Irr)
  Demux2/61 -> Subsystem2/2(Irr1)
  Demux2/62 -> Subsystem2/3(Irr2)
  Demux2/63 -> Subsystem2/4(Irr3)
  Demux2/64 -> Subsystem2/5(Irr4)
  Demux2/65 -> Subsystem2/6(Irr5)
  Demux2/66 -> Subsystem2/7(Irr6)
  Demux2/67 -> Subsystem3/1(Irr)
  Demux2/68 -> Subsystem3/2(Irr1)
  Demux2/69 -> Subsystem3/3(Irr2)
  Demux2/70 -> Subsystem3/4(Irr3)
  Demux2/71 -> Subsystem3/5(Irr4)
  Demux2/72 -> Subsystem3/6(Irr5)
  Demux2/73 -> Subsystem3/7(Irr6)
  Demux2/74 -> Subsystem4/1(Irr)
  Demux2/75 -> Subsystem4/2(Irr1)
  Demux2/76 -> Subsystem4/3(Irr2)
  Demux2/77 -> Subsystem4/4(Irr3)
  Demux2/78 -> Subsystem4/5(Irr4)
  Demux2/79 -> Subsystem4/6(Irr5)
  Demux2/80 -> Subsystem4/7(Irr6)
  Demux2/81 -> Subsystem5/1(Irr)
  Demux2/82 -> Subsystem5/2(Irr1)
  Demux2/83 -> Subsystem5/3(Irr2)
  Demux2/84 -> Subsystem5/4(Irr3)
  Demux2/85 -> Subsystem5/5(Irr4)
  Demux2/86 -> Subsystem5/6(Irr5)
  Demux2/87 -> Subsystem5/7(Irr6)
  Demux2/88 -> Subsystem6/1(Irr)
  Demux2/89 -> Subsystem6/2(Irr1)
  Demux2/90 -> Subsystem6/3(Irr2)
  Demux2/91 -> Subsystem6/4(Irr3)
  Demux2/92 -> Subsystem6/5(Irr4)
  Demux2/93 -> Subsystem6/6(Irr5)
  Demux2/94 -> Subsystem6/7(Irr6)
  Demux2/95 -> Subsystem7/1(Irr)
  Demux2/96 -> Subsystem7/2(Irr1)
  Demux2/97 -> Subsystem7/3(Irr2)
  Demux2/98 -> Subsystem7/4(Irr3)
  Demux2/99 -> Subsystem7/5(Irr4)
  Demux2/100 -> Subsystem7/6(Irr5)
  Demux2/101 -> Subsystem7/7(Irr6)
  Demux2/102 -> Subsystem8/1(Irr)
  Demux2/103 -> Subsystem8/2(Irr1)
  Demux2/104 -> Subsystem8/3(Irr2)
  Demux2/105 -> Subsystem8/4(Irr3)
  Demux2/106 -> Subsystem8/5(Irr4)
  Demux2/107 -> Subsystem8/6(Irr5)
  Demux2/108 -> Subsystem8/7(Irr6)
  Demux2/109 -> Subsystem9/1(Irr)
  Demux2/110 -> Subsystem9/2(Irr1)
  Demux2/111 -> Subsystem9/3(Irr2)
  Demux2/112 -> Subsystem9/4(Irr3)
  Demux2/113 -> Subsystem9/5(Irr4)
  Demux2/114 -> Subsystem9/6(Irr5)
  Demux2/115 -> Subsystem9/7(Irr6)
  Demux2/116 -> Subsystem10/1(Irr)
  Demux2/117 -> Subsystem10/2(Irr1)
  Demux2/118 -> Subsystem10/3(Irr2)
  Demux2/119 -> Subsystem10/4(Irr3)
  Demux2/120 -> Subsystem11/1(Irr)
  Demux2/121 -> Subsystem11/2(Irr1)
  connections:
  Variable DC Source1/LConn1 -- I1/RConn1 -- V1/LConn1
  Subsystem11/RConn1 -- Variable DC Source1/LConn2 -- V1/LConn2 -- Bypass Diode 11/LConn1
  Bypass Diode 21/RConn1 -- I1/LConn1 -- Subsystem21/LConn1
  Bypass Diode 22/RConn1 -- Subsystem21/RConn1 -- Bypass Diode 21/LConn1 -- Subsystem22/LConn1
  Subsystem23/LConn1 -- Subsystem22/RConn1 -- Bypass Diode 22/LConn1 -- Bypass Diode 23/RConn1
  Subsystem24/LConn1 -- Subsystem23/RConn1 -- Bypass Diode 23/LConn1 -- Bypass Diode 24/RConn1
  Subsystem29/LConn1 -- Bypass Diode 29/RConn1 -- Bypass Diode 24/LConn1 -- Subsystem24/RConn1
  Subsystem25/LConn1 -- Bypass Diode 29/LConn1 -- Subsystem29/RConn1 -- Bypass Diode 25/RConn1
  Subsystem27/LConn1 -- Bypass Diode 25/LConn1 -- Subsystem25/RConn1 -- Bypass Diode 27/RConn1
  Subsystem26/LConn1 -- Bypass Diode 27/LConn1 -- Subsystem27/RConn1 -- Bypass Diode 26/RConn1
  Subsystem28/LConn1 -- Subsystem26/RConn1 -- Bypass Diode 26/LConn1 -- Bypass Diode 28/RConn1
  Subsystem30/LConn1 -- Bypass Diode 28/LConn1 -- Subsystem28/RConn1 -- Bypass Diode 30/RConn1
  Bypass Diode 31/RConn1 -- Subsystem30/RConn1 -- Bypass Diode 30/LConn1 -- Subsystem31/LConn1
  Subsystem32/LConn1 -- Subsystem31/RConn1 -- Bypass Diode 31/LConn1 -- Bypass Diode 32/RConn1
  Subsystem33/LConn1 -- Bypass Diode 32/LConn1 -- Subsystem32/RConn1 -- Bypass Diode 33/RConn1
  Subsystem1/LConn1 -- Bypass Diode 33/LConn1 -- Subsystem33/RConn1 -- Bypass Diode 1/RConn1
  Subsystem2/LConn1 -- Subsystem1/RConn1 -- Bypass Diode 1/LConn1 -- Bypass Diode 2/RConn1
  Subsystem3/LConn1 -- Bypass Diode 2/LConn1 -- Subsystem2/RConn1 -- Bypass Diode 3/RConn1
  Bypass Diode 3/LConn1 -- Subsystem3/RConn1 -- Bypass Diode 4/RConn1 -- Subsystem4/LConn1
  Subsystem5/LConn1 -- Bypass Diode 5/RConn1 -- Subsystem4/RConn1 -- Bypass Diode 4/LConn1
  Subsystem6/LConn1 -- Subsystem5/RConn1 -- Bypass Diode 5/LConn1 -- Bypass Diode 6/RConn1
  Subsystem6/RConn1 -- Subsystem7/LConn1 -- Bypass Diode 7/RConn1 -- Bypass Diode 6/LConn1
  Bypass Diode 7/LConn1 -- Subsystem7/RConn1 -- Bypass Diode 8/RConn1 -- Subsystem8/LConn1
  Subsystem9/LConn1 -- Bypass Diode 8/LConn1 -- Subsystem8/RConn1 -- Bypass Diode 9/RConn1
  Subsystem10/LConn1 -- Bypass Diode 9/LConn1 -- Subsystem9/RConn1 -- Bypass Diode 10/RConn1
  Subsystem11/LConn1 -- Subsystem10/RConn1 -- Bypass Diode 10/LConn1 -- Bypass Diode 11/RConn1

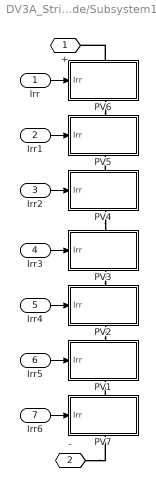
== system DV3A_String1_Diode/Subsystem1 ==
  Irr : Inport
  Irr1 : Inport  Port=2
  Irr2 : Inport  Port=3
  Irr3 : Inport  Port=4
  Irr4 : Inport  Port=5
  Irr5 : Inport  Port=6
  Irr6 : Inport  Port=7
  PV1 : Subsystem
      settings: PortSchema="{\"entries\":[{\"content\":{\"sides\":[{\"content\":{\"connectorIds\":[\"In1\"]},\"type\":\"ConnectorPlacement.EquallySpacedRectSide\",\"uuid\":\"5c508248-bd07-48d5-951d-be180bcc8740\"},{\"content\":{\"connectorIds\":[],\"side\":\"RIGHT\"},\"type\":\"ConnectorPlacement.EquallySpacedRectSide\",\"uuid\":\"e31a9bdc-b533-497f-8610-a92a4eef02bc\"},{\"content\":{\"connectorIds\":[\"LConn1\"],\"side\":\"TOP\"},\"type\":\"ConnectorPlacement.EquallySpacedRectSide\",\"uuid\":\"a80efd6c-0c74-41ec-a161-3d709011a457\"},{\"content\":{\"connectorIds\":[\"RConn1\"],\"side\":\"BOTTOM\"},\"type\":\"ConnectorPlacement.EquallySpacedRectSide\",\"uuid\":\"e2d028a7-872a-45fc-84e4-cb840db01281\"}]},\"type\":\"ConnectorPlacement.EquallySpacedConnector\",\"uuid\":\"57d442c0-d58c-4dd4-aeba-72d113e063d7\"}],\"packageUris\":[\"http://schema.mathworks.com/mf0/Connector/19700101\"],\"version\":\"1.0\"}"
  PV2 : Subsystem
      settings: PortSchema="{\"entries\":[{\"content\":{\"sides\":[{\"content\":{\"connectorIds\":[\"In1\"]},\"type\":\"ConnectorPlacement.EquallySpacedRectSide\",\"uuid\":\"5c508248-bd07-48d5-951d-be180bcc8740\"},{\"content\":{\"connectorIds\":[],\"side\":\"RIGHT\"},\"type\":\"ConnectorPlacement.EquallySpacedRectSide\",\"uuid\":\"e31a9bdc-b533-497f-8610-a92a4eef02bc\"},{\"content\":{\"connectorIds\":[\"LConn1\"],\"side\":\"TOP\"},\"type\":\"ConnectorPlacement.EquallySpacedRectSide\",\"uuid\":\"a80efd6c-0c74-41ec-a161-3d709011a457\"},{\"content\":{\"connectorIds\":[\"RConn1\"],\"side\":\"BOTTOM\"},\"type\":\"ConnectorPlacement.EquallySpacedRectSide\",\"uuid\":\"e2d028a7-872a-45fc-84e4-cb840db01281\"}]},\"type\":\"ConnectorPlacement.EquallySpacedConnector\",\"uuid\":\"57d442c0-d58c-4dd4-aeba-72d113e063d7\"}],\"packageUris\":[\"http://schema.mathworks.com/mf0/Connector/19700101\"],\"version\":\"1.0\"}"
  PV3 : Subsystem
      settings: PortSchema="{\"entries\":[{\"content\":{\"sides\":[{\"content\":{\"connectorIds\":[\"In1\"]},\"type\":\"ConnectorPlacement.EquallySpacedRectSide\",\"uuid\":\"5c508248-bd07-48d5-951d-be180bcc8740\"},{\"content\":{\"connectorIds\":[],\"side\":\"RIGHT\"},\"type\":\"ConnectorPlacement.EquallySpacedRectSide\",\"uuid\":\"e31a9bdc-b533-497f-8610-a92a4eef02bc\"},{\"content\":{\"connectorIds\":[\"LConn1\"],\"side\":\"TOP\"},\"type\":\"ConnectorPlacement.EquallySpacedRectSide\",\"uuid\":\"a80efd6c-0c74-41ec-a161-3d709011a457\"},{\"content\":{\"connectorIds\":[\"RConn1\"],\"side\":\"BOTTOM\"},\"type\":\"ConnectorPlacement.EquallySpacedRectSide\",\"uuid\":\"e2d028a7-872a-45fc-84e4-cb840db01281\"}]},\"type\":\"ConnectorPlacement.EquallySpacedConnector\",\"uuid\":\"57d442c0-d58c-4dd4-aeba-72d113e063d7\"}],\"packageUris\":[\"http://schema.mathworks.com/mf0/Connector/19700101\"],\"version\":\"1.0\"}"
  PV4 : Subsystem
      settings: PortSchema="{\"entries\":[{\"content\":{\"sides\":[{\"content\":{\"connectorIds\":[\"In1\"]},\"type\":\"ConnectorPlacement.EquallySpacedRectSide\",\"uuid\":\"5c508248-bd07-48d5-951d-be180bcc8740\"},{\"content\":{\"connectorIds\":[],\"side\":\"RIGHT\"},\"type\":\"ConnectorPlacement.EquallySpacedRectSide\",\"uuid\":\"e31a9bdc-b533-497f-8610-a92a4eef02bc\"},{\"content\":{\"connectorIds\":[\"LConn1\"],\"side\":\"TOP\"},\"type\":\"ConnectorPlacement.EquallySpacedRectSide\",\"uuid\":\"a80efd6c-0c74-41ec-a161-3d709011a457\"},{\"content\":{\"connectorIds\":[\"RConn1\"],\"side\":\"BOTTOM\"},\"type\":\"ConnectorPlacement.EquallySpacedRectSide\",\"uuid\":\"e2d028a7-872a-45fc-84e4-cb840db01281\"}]},\"type\":\"ConnectorPlacement.EquallySpacedConnector\",\"uuid\":\"57d442c0-d58c-4dd4-aeba-72d113e063d7\"}],\"packageUris\":[\"http://schema.mathworks.com/mf0/Connector/19700101\"],\"version\":\"1.0\"}"
  PV5 : Subsystem
      settings: PortSchema="{\"entries\":[{\"content\":{\"sides\":[{\"content\":{\"connectorIds\":[\"In1\"]},\"type\":\"ConnectorPlacement.EquallySpacedRectSide\",\"uuid\":\"5c508248-bd07-48d5-951d-be180bcc8740\"},{\"content\":{\"connectorIds\":[],\"side\":\"RIGHT\"},\"type\":\"ConnectorPlacement.EquallySpacedRectSide\",\"uuid\":\"e31a9bdc-b533-497f-8610-a92a4eef02bc\"},{\"content\":{\"connectorIds\":[\"LConn1\"],\"side\":\"TOP\"},\"type\":\"ConnectorPlacement.EquallySpacedRectSide\",\"uuid\":\"a80efd6c-0c74-41ec-a161-3d709011a457\"},{\"content\":{\"connectorIds\":[\"RConn1\"],\"side\":\"BOTTOM\"},\"type\":\"ConnectorPlacement.EquallySpacedRectSide\",\"uuid\":\"e2d028a7-872a-45fc-84e4-cb840db01281\"}]},\"type\":\"ConnectorPlacement.EquallySpacedConnector\",\"uuid\":\"57d442c0-d58c-4dd4-aeba-72d113e063d7\"}],\"packageUris\":[\"http://schema.mathworks.com/mf0/Connector/19700101\"],\"version\":\"1.0\"}"
  PV6 : Subsystem
      settings: PortSchema="{\"entries\":[{\"content\":{\"sides\":[{\"content\":{\"connectorIds\":[\"In1\"]},\"type\":\"ConnectorPlacement.EquallySpacedRectSide\",\"uuid\":\"5c508248-bd07-48d5-951d-be180bcc8740\"},{\"content\":{\"connectorIds\":[],\"side\":\"RIGHT\"},\"type\":\"ConnectorPlacement.EquallySpacedRectSide\",\"uuid\":\"e31a9bdc-b533-497f-8610-a92a4eef02bc\"},{\"content\":{\"connectorIds\":[\"LConn1\"],\"side\":\"TOP\"},\"type\":\"ConnectorPlacement.EquallySpacedRectSide\",\"uuid\":\"a80efd6c-0c74-41ec-a161-3d709011a457\"},{\"content\":{\"connectorIds\":[\"RConn1\"],\"side\":\"BOTTOM\"},\"type\":\"ConnectorPlacement.EquallySpacedRectSide\",\"uuid\":\"e2d028a7-872a-45fc-84e4-cb840db01281\"}]},\"type\":\"ConnectorPlacement.EquallySpacedConnector\",\"uuid\":\"57d442c0-d58c-4dd4-aeba-72d113e063d7\"}],\"packageUris\":[\"http://schema.mathworks.com/mf0/Connector/19700101\"],\"version\":\"1.0\"}"
  PV7 : Subsystem
      settings: PortSchema="{\"entries\":[{\"content\":{\"sides\":[{\"content\":{\"connectorIds\":[\"In1\"]},\"type\":\"ConnectorPlacement.EquallySpacedRectSide\",\"uuid\":\"5c508248-bd07-48d5-951d-be180bcc8740\"},{\"content\":{\"connectorIds\":[],\"side\":\"RIGHT\"},\"type\":\"ConnectorPlacement.EquallySpacedRectSide\",\"uuid\":\"e31a9bdc-b533-497f-8610-a92a4eef02bc\"},{\"content\":{\"connectorIds\":[\"LConn1\"],\"side\":\"TOP\"},\"type\":\"ConnectorPlacement.EquallySpacedRectSide\",\"uuid\":\"a80efd6c-0c74-41ec-a161-3d709011a457\"},{\"content\":{\"connectorIds\":[\"RConn1\"],\"side\":\"BOTTOM\"},\"type\":\"ConnectorPlacement.EquallySpacedRectSide\",\"uuid\":\"e2d028a7-872a-45fc-84e4-cb840db01281\"}]},\"type\":\"ConnectorPlacement.EquallySpacedConnector\",\"uuid\":\"57d442c0-d58c-4dd4-aeba-72d113e063d7\"}],\"packageUris\":[\"http://schema.mathworks.com/mf0/Connector/19700101\"],\"version\":\"1.0\"}"
  + : PMIOPort  Side=Left
  - : PMIOPort  Port=2  Side=Right
  wires:
  Irr2/1 -> PV4/1(Irr)
  Irr/1 -> PV6/1(Irr)
  Irr1/1 -> PV5/1(Irr)
  Irr3/1 -> PV3/1(Irr)
  Irr5/1 -> PV1/1(Irr)
  Irr4/1 -> PV2/1(Irr)
  Irr6/1 -> PV7/1(Irr)
  connections:
  PV6/LConn1 -- +/RConn1
  PV4/LConn1 -- PV5/RConn1
  PV6/RConn1 -- PV5/LConn1
  PV3/RConn1 -- PV2/LConn1
  PV2/RConn1 -- PV1/LConn1
  PV4/RConn1 -- PV3/LConn1
  -/RConn1 -- PV7/RConn1
  PV7/LConn1 -- PV1/RConn1

== system DV3A_String1_Diode/Subsystem10 ==
  Irr : Inport
  Irr1 : Inport  Port=2
  Irr2 : Inport  Port=3
  Irr3 : Inport  Port=4
  PV1 : Subsystem
      settings: PortSchema="{\"entries\":[{\"content\":{\"sides\":[{\"content\":{\"connectorIds\":[\"In1\"]},\"type\":\"ConnectorPlacement.EquallySpacedRectSide\",\"uuid\":\"5c508248-bd07-48d5-951d-be180bcc8740\"},{\"content\":{\"connectorIds\":[],\"side\":\"RIGHT\"},\"type\":\"ConnectorPlacement.EquallySpacedRectSide\",\"uuid\":\"e31a9bdc-b533-497f-8610-a92a4eef02bc\"},{\"content\":{\"connectorIds\":[\"LConn1\"],\"side\":\"TOP\"},\"type\":\"ConnectorPlacement.EquallySpacedRectSide\",\"uuid\":\"a80efd6c-0c74-41ec-a161-3d709011a457\"},{\"content\":{\"connectorIds\":[\"RConn1\"],\"side\":\"BOTTOM\"},\"type\":\"ConnectorPlacement.EquallySpacedRectSide\",\"uuid\":\"e2d028a7-872a-45fc-84e4-cb840db01281\"}]},\"type\":\"ConnectorPlacement.EquallySpacedConnector\",\"uuid\":\"57d442c0-d58c-4dd4-aeba-72d113e063d7\"}],\"packageUris\":[\"http://schema.mathworks.com/mf0/Connector/19700101\"],\"version\":\"1.0\"}"
  PV2 : Subsystem
      settings: PortSchema="{\"entries\":[{\"content\":{\"sides\":[{\"content\":{\"connectorIds\":[\"In1\"]},\"type\":\"ConnectorPlacement.EquallySpacedRectSide\",\"uuid\":\"5c508248-bd07-48d5-951d-be180bcc8740\"},{\"content\":{\"connectorIds\":[],\"side\":\"RIGHT\"},\"type\":\"ConnectorPlacement.EquallySpacedRectSide\",\"uuid\":\"e31a9bdc-b533-497f-8610-a92a4eef02bc\"},{\"content\":{\"connectorIds\":[\"LConn1\"],\"side\":\"TOP\"},\"type\":\"ConnectorPlacement.EquallySpacedRectSide\",\"uuid\":\"a80efd6c-0c74-41ec-a161-3d709011a457\"},{\"content\":{\"connectorIds\":[\"RConn1\"],\"side\":\"BOTTOM\"},\"type\":\"ConnectorPlacement.EquallySpacedRectSide\",\"uuid\":\"e2d028a7-872a-45fc-84e4-cb840db01281\"}]},\"type\":\"ConnectorPlacement.EquallySpacedConnector\",\"uuid\":\"57d442c0-d58c-4dd4-aeba-72d113e063d7\"}],\"packageUris\":[\"http://schema.mathworks.com/mf0/Connector/19700101\"],\"version\":\"1.0\"}"
  PV3 : Subsystem
      settings: PortSchema="{\"entries\":[{\"content\":{\"sides\":[{\"content\":{\"connectorIds\":[\"In1\"]},\"type\":\"ConnectorPlacement.EquallySpacedRectSide\",\"uuid\":\"5c508248-bd07-48d5-951d-be180bcc8740\"},{\"content\":{\"connectorIds\":[],\"side\":\"RIGHT\"},\"type\":\"ConnectorPlacement.EquallySpacedRectSide\",\"uuid\":\"e31a9bdc-b533-497f-8610-a92a4eef02bc\"},{\"content\":{\"connectorIds\":[\"LConn1\"],\"side\":\"TOP\"},\"type\":\"ConnectorPlacement.EquallySpacedRectSide\",\"uuid\":\"a80efd6c-0c74-41ec-a161-3d709011a457\"},{\"content\":{\"connectorIds\":[\"RConn1\"],\"side\":\"BOTTOM\"},\"type\":\"ConnectorPlacement.EquallySpacedRectSide\",\"uuid\":\"e2d028a7-872a-45fc-84e4-cb840db01281\"}]},\"type\":\"ConnectorPlacement.EquallySpacedConnector\",\"uuid\":\"57d442c0-d58c-4dd4-aeba-72d113e063d7\"}],\"packageUris\":[\"http://schema.mathworks.com/mf0/Connector/19700101\"],\"version\":\"1.0\"}"
  PV4 : Subsystem
      settings: PortSchema="{\"entries\":[{\"content\":{\"sides\":[{\"content\":{\"connectorIds\":[\"In1\"]},\"type\":\"ConnectorPlacement.EquallySpacedRectSide\",\"uuid\":\"5c508248-bd07-48d5-951d-be180bcc8740\"},{\"content\":{\"connectorIds\":[],\"side\":\"RIGHT\"},\"type\":\"ConnectorPlacement.EquallySpacedRectSide\",\"uuid\":\"e31a9bdc-b533-497f-8610-a92a4eef02bc\"},{\"content\":{\"connectorIds\":[\"LConn1\"],\"side\":\"TOP\"},\"type\":\"ConnectorPlacement.EquallySpacedRectSide\",\"uuid\":\"a80efd6c-0c74-41ec-a161-3d709011a457\"},{\"content\":{\"connectorIds\":[\"RConn1\"],\"side\":\"BOTTOM\"},\"type\":\"ConnectorPlacement.EquallySpacedRectSide\",\"uuid\":\"e2d028a7-872a-45fc-84e4-cb840db01281\"}]},\"type\":\"ConnectorPlacement.EquallySpacedConnector\",\"uuid\":\"57d442c0-d58c-4dd4-aeba-72d113e063d7\"}],\"packageUris\":[\"http://schema.mathworks.com/mf0/Connector/19700101\"],\"version\":\"1.0\"}"
  + : PMIOPort  Side=Left
  - : PMIOPort  Port=2  Side=Right
  wires:
  Irr2/1 -> PV1/1(Irr)
  Irr/1 -> PV2/1(Irr)
  Irr1/1 -> PV4/1(Irr)
  Irr3/1 -> PV3/1(Irr)
  connections:
  PV2/LConn1 -- +/RConn1
  PV4/RConn1 -- PV1/LConn1
  PV4/LConn1 -- PV2/RConn1
  PV3/RConn1 -- -/RConn1
  PV1/RConn1 -- PV3/LConn1

== system DV3A_String1_Diode/Subsystem11 ==
  Irr : Inport
  Irr1 : Inport  Port=2
  PV1 : Subsystem
      settings: PortSchema="{\"entries\":[{\"content\":{\"sides\":[{\"content\":{\"connectorIds\":[\"In1\"]},\"type\":\"ConnectorPlacement.EquallySpacedRectSide\",\"uuid\":\"5c508248-bd07-48d5-951d-be180bcc8740\"},{\"content\":{\"connectorIds\":[],\"side\":\"RIGHT\"},\"type\":\"ConnectorPlacement.EquallySpacedRectSide\",\"uuid\":\"e31a9bdc-b533-497f-8610-a92a4eef02bc\"},{\"content\":{\"connectorIds\":[\"LConn1\"],\"side\":\"TOP\"},\"type\":\"ConnectorPlacement.EquallySpacedRectSide\",\"uuid\":\"a80efd6c-0c74-41ec-a161-3d709011a457\"},{\"content\":{\"connectorIds\":[\"RConn1\"],\"side\":\"BOTTOM\"},\"type\":\"ConnectorPlacement.EquallySpacedRectSide\",\"uuid\":\"e2d028a7-872a-45fc-84e4-cb840db01281\"}]},\"type\":\"ConnectorPlacement.EquallySpacedConnector\",\"uuid\":\"57d442c0-d58c-4dd4-aeba-72d113e063d7\"}],\"packageUris\":[\"http://schema.mathworks.com/mf0/Connector/19700101\"],\"version\":\"1.0\"}"
  PV10 : Subsystem
      settings: PortSchema="{\"entries\":[{\"content\":{\"sides\":[{\"content\":{\"connectorIds\":[\"In1\"]},\"type\":\"ConnectorPlacement.EquallySpacedRectSide\",\"uuid\":\"5c508248-bd07-48d5-951d-be180bcc8740\"},{\"content\":{\"connectorIds\":[],\"side\":\"RIGHT\"},\"type\":\"ConnectorPlacement.EquallySpacedRectSide\",\"uuid\":\"e31a9bdc-b533-497f-8610-a92a4eef02bc\"},{\"content\":{\"connectorIds\":[\"LConn1\"],\"side\":\"TOP\"},\"type\":\"ConnectorPlacement.EquallySpacedRectSide\",\"uuid\":\"a80efd6c-0c74-41ec-a161-3d709011a457\"},{\"content\":{\"connectorIds\":[\"RConn1\"],\"side\":\"BOTTOM\"},\"type\":\"ConnectorPlacement.EquallySpacedRectSide\",\"uuid\":\"e2d028a7-872a-45fc-84e4-cb840db01281\"}]},\"type\":\"ConnectorPlacement.EquallySpacedConnector\",\"uuid\":\"57d442c0-d58c-4dd4-aeba-72d113e063d7\"}],\"packageUris\":[\"http://schema.mathworks.com/mf0/Connector/19700101\"],\"version\":\"1.0\"}"
  + : PMIOPort  Side=Left
  - : PMIOPort  Port=2  Side=Right
  wires:
  Irr/1 -> PV10/1(Irr)
  Irr1/1 -> PV1/1(Irr)
  connections:
  PV10/LConn1 -- +/RConn1
  PV1/RConn1 -- -/RConn1
  PV10/RConn1 -- PV1/LConn1
